simulink model "rocket_prop_eval"  (R2020b)
settings: Solver=VariableStepAuto  StartTime=0.0  StopTime=100  RelTol=1e-3
libraries: simulink x2, shared3dof x1, pid_lib x1
settings Model: Creator=Hariharan  LastModifiedBy=Hariharan

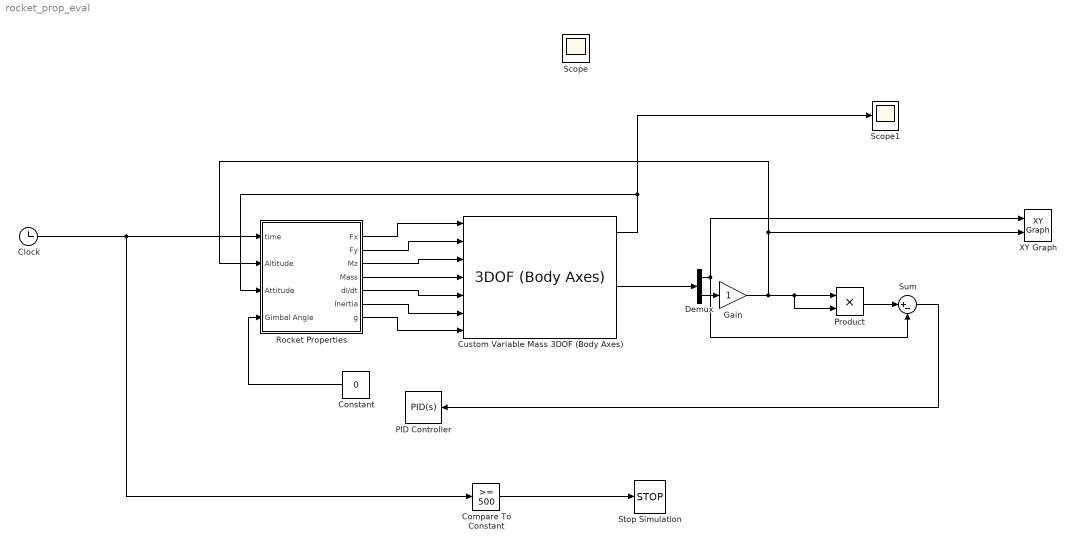
== system rocket_prop_eval ==
  Clock : Clock
  Compare To Constant : simulink/Logic and Bit Operations/Compare To Constant  relop=>=  const=500  OutDataTypeStr=boolean
  Constant : Constant  Value=0
  Custom Variable Mass 3DOF (Body Axes) : shared3dof/3DOF (Body Axes)  units=Metric (MKS)  mtype=Custom Variable  v_ini=0  theta_ini=0  alpha_ini=0  pos_ini=[0 0]  q_ini=0  mass=1.0  mass_e=0.5  mass_f=3.0  Iyy=1.0  Iyy_e=0.5  Iyy_f=3.0  g_in=External  g=9.81  vre_flag=off  abi_flag=off  aMode=0  vel_statename=''  theta_statename=''  pos_statename=''  q_statename=''  mass_statename=''
      settings: SourceProductBaseCode=AE,PW,MT,UV,VE,VP
  Demux : Demux  Outputs=2
  Gain : Gain
  PID Controller : pid_lib/PID Controller  Controller=PID  Form=Parallel  TimeDomain=Continuous-time  UseExternalTs=off  SampleTime=-1  IntegratorMethod=Forward Euler  FilterMethod=Forward Euler  ControllerParametersSource=internal  P=0.01  I=1  D=0.1  UseFilter=on  N=100  TunerSelectOption=Transfer Function Based (PID Tuner App)  InitialConditionSource=internal  InitialConditionForIntegrator=0  InitialConditionForFilter=0  DifferentiatorICPrevScaledInput=0  ExternalReset=none  TrackingMode=off  Kt=1  LimitOutput=off  SatLimitsSource=internal  UpperSaturationLimit=inf  LowerSaturationLimit=-inf  LinearizeAsGain=on  AntiWindupMode=none  Kb=1  POutMin=[]  POutMax=[]  IOutMin=[]  IOutMax=[]  DOutMin=[]  DOutMax=[]  NOutMin=[]  NOutMax=[]  SumOutMin=[]  SumOutMax=[]  SaturationOutMin=[]  SaturationOutMax=[]  PParamMin=[]  PParamMax=[]  IParamMin=[]  IParamMax=[]  DParamMin=[]  DParamMax=[]  NParamMin=[]  NParamMax=[]  KbParamMin=[]  KbParamMax=[]  KtParamMin=[]  KtParamMax=[]  KbOutMin=[]  KbOutMax=[]  KtOutMin=[]  KtOutMax=[]  IntegratorOutMin=[]  IntegratorOutMax=[]  FilterOutMin=[]  FilterOutMax=[]  SumI1OutMin=[]  SumI1OutMax=[]  SumI2OutMin=[]  SumI2OutMax=[]  SumI3OutMin=[]  SumI3OutMax=[]  SumI4OutMin=[]  SumI4OutMax=[]  SumDOutMin=[]  SumDOutMax=[]  DifferentiatorOutMin=[]  DifferentiatorOutMax=[]  FilterDiffOutCoefMin=[]  FilterDiffOutCoefMax=[]  ReciprocalOutMin=[]  ReciprocalOutMax=[]  SumDenOutMin=[]  SumDenOutMax=[]  SumNumOutMin=[]  SumNumOutMax=[]  DivideOutMin=[]  DivideOutMax=[]  UdiffTsProdOutMin=[]  UdiffTsProdOutMax=[]  NTsProdOutMin=[]  NTsProdOutMax=[]  UintegralTsProdOutMin=[]  UintegralTsProdOutMax=[]  UngainTsProdOutMin=[]  UngainTsProdOutMax=[]  IntegratorContinuousStateAttributes=''  IntegratorStateMustResolveToSignalObject=off  IntegratorRTWStateStorageClass=Auto  FilterContinuousStateAttributes=''  FilterStateMustResolveToSignalObject=off  FilterRTWStateStorageClass=Auto  ParallelPVariant=InternalParameters  IdealPVariant=Disabled  IVariant=InternalParameters  DVariant=InternalParameters  IntegratorVariant=Continuous  SatVariant=Disabled  AWVariant=Passthrough  PCopyVariant=Disabled  TRVariant=Disabled  FdbkBlocksVariant=Forward  IdealPFdbkVariant=Disabled  SatFdbkVariant=Disabled  DerivativeFilterVariant=ContFilter  NVariant=InternalParameters  NCopyVariant=Disabled  FilterICVariant=InternalICsFilter  IntegratorICVariant=InternalICs  ExternalResetVariant=Disabled  TRSumVariant=Passthrough  SumFdbkVariant=Disabled  SumVariant=Sum_PID  TsampFilterVariant=InternalTs  TsampNgainVariant=Passthrough  TsampIntegralVariant=Passthrough  ExternalSaturationOutDataTypeStr=Inherit: Same as second input
  Product : Product
  Rocket Properties : Subsystem
  Scope : Scope
  Scope1 : Scope
  Stop Simulation : Stop
  Sum : Sum  Inputs=|+-
  XY Graph : simulink/Sinks/XY Graph  xmin=0  xmax=1000  ymin=0  ymax=5000  st=-1
  wires:
  Rocket Properties/1(Fx) -> Custom Variable Mass 3DOF (Body Axes)/1
  Rocket Properties/2(Fy) -> Custom Variable Mass 3DOF (Body Axes)/2
  Rocket Properties/3(Mz) -> Custom Variable Mass 3DOF (Body Axes)/3
  Rocket Properties/4(Mass) -> Custom Variable Mass 3DOF (Body Axes)/4
  Rocket Properties/5(dI/dt) -> Custom Variable Mass 3DOF (Body Axes)/5
  Rocket Properties/6(Inertia) -> Custom Variable Mass 3DOF (Body Axes)/6
  Clock/1 -> Compare To Constant/1, Rocket Properties/1(time)
  Custom Variable Mass 3DOF (Body Axes)/4 -> Demux/1
  Demux/2 -> Gain/1
  Gain/1 -> Product/2, Product/1, XY Graph/2, Rocket Properties/2(Altitude)
  Custom Variable Mass 3DOF (Body Axes)/1 -> Scope1/1, Rocket Properties/3(Attitude)
  Product/1 -> Sum/1
  Demux/1 -> Sum/2, XY Graph/1
  Sum/1 -> PID Controller/1
  Compare To Constant/1 -> Stop Simulation/1
  Constant/1 -> Rocket Properties/4(Gimbal Angle)
  Rocket Properties/7(g) -> Custom Variable Mass 3DOF (Body Axes)/7

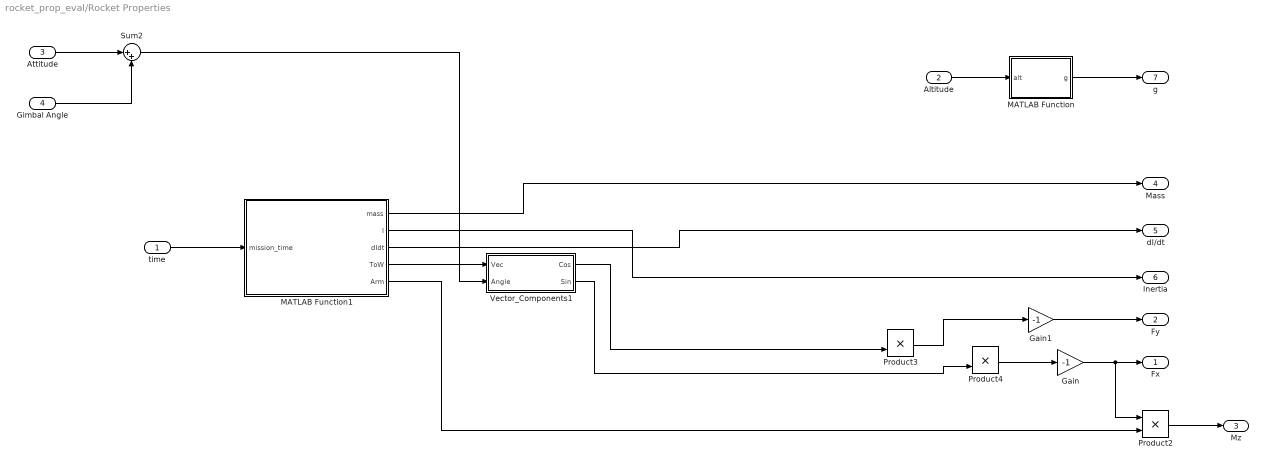
== system rocket_prop_eval/Rocket Properties ==
  time : Inport
  Altitude : Inport  Port=2
  Attitude : Inport  Port=3
  Gimbal Angle : Inport  Port=4
  Gain : Gain  Gain=-1
  Gain1 : Gain  Gain=-1
  MATLAB Function : MATLAB Function  TreatAsAtomicUnit=on
  MATLAB Function1 : MATLAB Function  TreatAsAtomicUnit=on
  Product2 : Product
  Product3 : Product
  Product4 : Product
  Sum2 : Sum  Inputs=|++
  Vector_Components1 : Subsystem
  Fx : Outport
  Fy : Outport  Port=2
  Mz : Outport  Port=3
  Mass : Outport  Port=4
  dI/dt : Outport  Port=5
  Inertia : Outport  Port=6
  g : Outport  Port=7
  wires:
  Altitude/1 -> MATLAB Function/1(alt)
  time/1 -> MATLAB Function1/1(mission_time)
  MATLAB Function1/3(dIdt) -> dI/dt/1
  MATLAB Function1/2(I) -> Inertia/1
  MATLAB Function1/1(mass) -> Mass/1
  MATLAB Function1/5(Arm) -> Product2/2
  Product2/1 -> Mz/1
  MATLAB Function1/4(ToW) -> Vector_Components1/1(Vec)
  Vector_Components1/1(Cos) -> Product3/2
  Vector_Components1/2(Sin) -> Product4/2
  Product4/1 -> Gain/1
  Product3/1 -> Gain1/1
  Attitude/1 -> Sum2/1
  Gimbal Angle/1 -> Sum2/2
  Sum2/1 -> Vector_Components1/2(Angle)
  Gain1/1 -> Fy/1
  Gain/1 -> Product2/1, Fx/1
  MATLAB Function/1(g) -> g/1

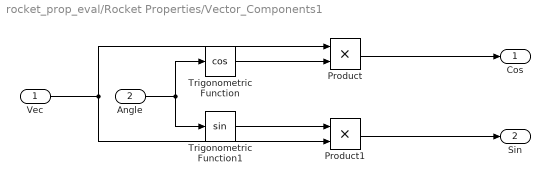
== system rocket_prop_eval/Rocket Properties/Vector_Components1 ==
  Vec : Inport
  Angle : Inport  Port=2
  Product : Product
  Product1 : Product
  Trigonometric Function : Trigonometry  Operator=cos
  Trigonometric Function1 : Trigonometry
  Cos : Outport
  Sin : Outport  Port=2
  wires:
  Vec/1 -> Product/1, Product1/2
  Trigonometric Function/1 -> Product/2
  Trigonometric Function1/1 -> Product1/1
  Angle/1 -> Trigonometric Function1/1, Trigonometric Function/1
  Product1/1 -> Sin/1
  Product/1 -> Cos/1

== matlab function rocket_prop_eval/Rocket Properties/MATLAB Function1 ==
  data: mission_time input; mass output; I output; dIdt output; ToW output; Arm output
function [mass,I,dIdt,ToW,Arm] = rocket_prop_eval(mission_time)

L = [14.52 1.95 1.83];

tbb = [114.8962  156.7683  261.4940];

m0 = [1.1112e4    0.1664e4    0.0239e4];

M0 = 1.3065e+04;

m_dot = [69.2893    7.4443    0.5640];

Diam = 0.83;

thick = 0.001;


if mission_time < tbb(1)
        
        m_dot_current = m_dot(1);
        
        mass = M0 - (m_dot(1)*mission_time);
        
        Length = sum(L);
        
        ToW = 2;
        
    elseif (mission_time >= tbb(1)) && (mission_time < sum(tbb(1:2)))
        
        m_dot_current = m_dot(2);
        
        mass = M0 - m0(1) - (m_dot(2)*(mission_time - tbb(1))); 
        
        Length = sum(L(2:end));
        
        ToW = 2;
        
    else
        
        m_dot_current = m_dot(3);
        
        mass = M0 - m0(1) - m0(2) - (m_dot(3)*(mission_time - tbb(1) - tbb(2)));
        
        Length = sum(L(end));
        
        ToW = 10000/mass;
        
end
    
I = 0.5*mass*(Diam/2)^2;

dIdt = m_dot_current;

Arm = Length/2;

end

== matlab function rocket_prop_eval/Rocket Properties/MATLAB Function ==
  data: alt input; g output
function g = g_calc(alt)

Mu = 3.986004418e14;
Re = 6.371e6;

R = Re + alt;

g = (Mu/(R^2));

end
